simulink model "DataCenterStability"  (R2025b)
settings: Solver=daessc  StartTime=0  StopTime=7  FixedStep=5e-5  MaxStep=0.001  RelTol=1e-3
PostLoadFcn:
  | DataCenterParamScan
InitFcn:
  | opFile_ = fullfile(fileparts(which('DataCenterStability')), 'DataCenterStability_SteadyStateOP.mat');
  | if isfile(opFile_)
  |     tmp_ = load(opFile_, 'op');
  |     assignin('base', 'ssOP__', tmp_.op);
  | end
  | warning('off','physmod:common:mf:system:xform:DelayUnsupportedWithOperatingPoint');
  | warning('off','physmod:common:mf:system:xform:TimeUnsupportedWithOperatingPoint');
values from neighbouring files (symbols this model uses):
  baseVoltageDC = ups.Vdc    [DataCenterParamScan.m]
  bessConverterEfficiency = ups.DCBus.converterEff    [DataCenterParamScan.m]
  droopGain = ups.DCBus.droop    [DataCenterParamScan.m]
  filterInductance = ups.inverter.filterInductance    [DataCenterParamScan.m]
  filterInductanceAFE = ups.AFE.filterInductance    [DataCenterParamScan.m]
  filterResistance = ups.inverter.filterResistance    [DataCenterParamScan.m]
  filterResistanceAFE = ups.AFE.filterResistance    [DataCenterParamScan.m]
  frequency = ups.frequency    [DataCenterParamScan.m]
  G1 = 1    [DataCenterParamScan.m]
  G2 = 0    [DataCenterParamScan.m]
  iBatt = ups.batt.iRated    [DataCenterParamScan.m]
  initialMode = ups.batt.initialMode    [DataCenterParamScan.m]
  invKiId = ups.inverter.kiId    [DataCenterParamScan.m]
  invKiVd = ups.inverter.kiVd    [DataCenterParamScan.m]
  invKpId = ups.inverter.kpId    [DataCenterParamScan.m]
  invKpVd = ups.inverter.kpVd    [DataCenterParamScan.m]
  kpDC = ups.DCBus.kpDC    [DataCenterParamScan.m]
  N_pfc = round(N_total * [1/3, 1/3, 1/3])    [DataCenterParamScan.m]    (also in StabilityStudy.m = cfg.Topology.N_pfc)
  plantRating = ups.rating    [DataCenterParamScan.m]
  powerTau = 0.005    [DataCenterParamScan.m]
  rampRate = ups.batt.rampRate    [DataCenterParamScan.m]
  scan = obj.Cfg.GNC    [GNCAnalyzer.m]
  Ts = 5e-5    (= 5e-05)    [DataCenterParamScan.m]
  Vac = ups.Vac    [DataCenterParamScan.m]
  vBattMax = ups.batt.VMax    [DataCenterParamScan.m]
  vBattNom = ups.batt.Vnom    [DataCenterParamScan.m]
  vDCThreshold = ups.DCBus.VThreshold    [DataCenterParamScan.m]
  vGridMin = ups.DCBus.gridThreshold    [DataCenterParamScan.m]
undefined symbols (not defined in the file or in its folder): ctLimitDelayTime, DiscIntNeverNeededParam, ee_sli_rtmsupport, gcbh, itTray, pfc, serverTray, ups
libraries: fl_lib x77, nesl_utility x35, ee_lib x30, simulink x17, eeGeneralControl x14, datacenter_lib x12, eeTransforms x7, slpidlib x4, nesl_utility_internal x4, simulink_extras x3, datacenterCompositeLib x2, eePowerMeasurement x2
(part 1 of 5)
settings Model: SimulationMode=accelerator  Creator=rajarshd  LastModifiedBy=rajarshd
settings SolverCC: AllowMultiTaskInputOutput=on  ZeroCrossAlgorithm=Adaptive  AutoInsertRateTranBlk=on
settings DataIOCC: FinalStateName=xFinal_ss  InitialState=xInitOP__  SaveOperatingPoint=on  SaveOutput=off  DSMLogging=off  SaveTime=off  StateSaveName=xoutState
settings DebuggingCC: InheritedTsInSrcMsg=none  MultiTaskRateTransMsg=warning
settings SimscapeCC: SimscapeNominalValues="[{\"value\":\"1\",\"unit\":\"A\"},{\"value\":\"1\",\"unit\":\"bar\"},{\"value\":\"1\",\"unit\":\"cm^2\"},{\"value\":\"1\",\"unit\":\"cm^3/s\"},{\"value\":\"1\",\"unit\":\"kJ/kg\"},{\"value\":\"1\",\"unit\":\"kW\"},{\"value\":\"1\",\"unit\":\"l\"},{\"value\":\"1\",\"unit\":\"N\"},{\"value\":\"1\",\"unit\":\"N*m\"},{\"value\":\"1\",\"unit\":\"V\"},{\"value\":\"0.001\",\"unit\":\"Wb\"}]"  SimscapeLogType=all  SimscapeLogDecimation=50.0  SimscapeLogLimitData=off  SimscapeLogDataHistory=10000.0  SimscapeUseOperatingPoints=on  SimscapeOperatingPoint=ssOP__  SimscapeCompileComponentReuse=on
settings ExplorerConfigSet: SimMechanicsOpenEditorOnUpdate=off

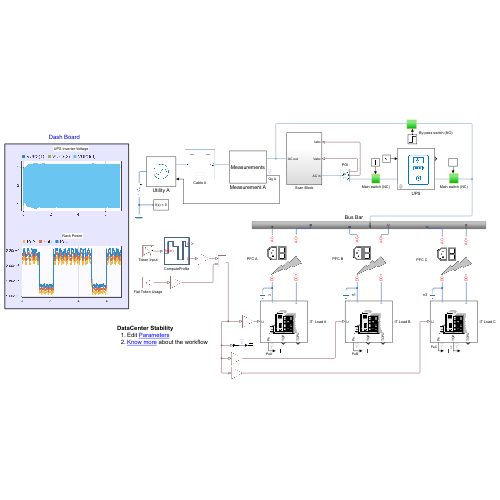
[thumbnail: Simulink's stored preview of the top-level diagram]
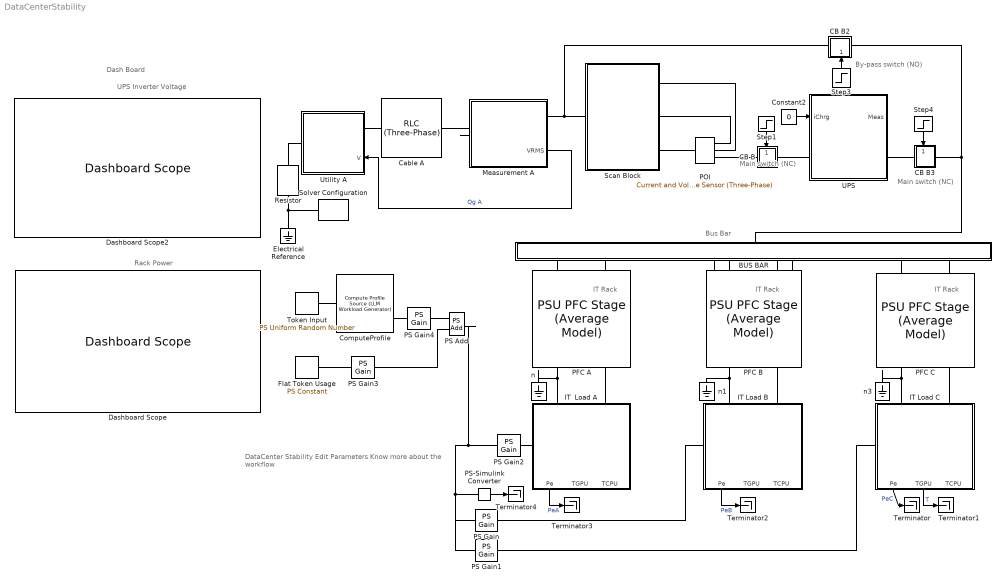
== system DataCenterStability ==
  note: DataCenter Stability
      | Edit Parameters
      | Know more about the workflow
  note: Dash Board
  note: By-pass switch (NO)
  note: Rack Power
  note: IT Rack
  note: IT Rack
  note: IT Rack
  note: Bus Bar
  note: Main switch (NC)
  note: Main switch (NC)
  note: UPS Inverter Voltage
  BUS BAR : Subsystem
  CB B : Subsystem
      settings: PortSchema="{\"entries\":[{\"content\":{\"sides\":[{\"content\":{\"connectorIds\":[\"In1\"]},\"type\":\"ConnectorPlacement.EquallySpacedRectSide\",\"uuid\":\"67c0f727-7c15-41c9-98df-b3c7d57498ed\"},{\"content\":{\"side\":\"RIGHT\"},\"type\":\"ConnectorPlacement.EquallySpacedRectSide\",\"uuid\":\"7fc39429-ba61-416d-b42b-93e81eb2f426\"},{\"content\":{\"connectorIds\":[\"LConn1\"],\"side\":\"TOP\"},\"type\":\"ConnectorPlacement.EquallySpacedRectSide\",\"uuid\":\"c6dd9263-b57a-4cff-a218-af99f2798f29\"},{\"content\":{\"connectorIds\":[\"RConn1\"],\"side\":\"BOTTOM\"},\"type\":\"ConnectorPlacement.EquallySpacedRectSide\",\"uuid\":\"e2a2ba44-d59d-4e27-adf1-3f94e828ca78\"}]},\"type\":\"ConnectorPlacement.EquallySpacedConnector\",\"uuid\":\"b349a99b-c902-4df9-9c99-34841afb28dd\"}],\"packageUris\":[\"http://schema.mathworks.com/mf0/Connector/R2020b\"],\"version\":\"1.0\"}"
  CB B2 : Subsystem
      settings: PortSchema="{\"entries\":[{\"content\":{\"sides\":[{\"content\":{},\"type\":\"ConnectorPlacement.EquallySpacedRectSide\",\"uuid\":\"67c0f727-7c15-41c9-98df-b3c7d57498ed\"},{\"content\":{\"connectorIds\":[\"In1\"],\"side\":\"RIGHT\"},\"type\":\"ConnectorPlacement.EquallySpacedRectSide\",\"uuid\":\"7fc39429-ba61-416d-b42b-93e81eb2f426\"},{\"content\":{\"connectorIds\":[\"LConn1\"],\"side\":\"TOP\"},\"type\":\"ConnectorPlacement.EquallySpacedRectSide\",\"uuid\":\"c6dd9263-b57a-4cff-a218-af99f2798f29\"},{\"content\":{\"connectorIds\":[\"RConn1\"],\"side\":\"BOTTOM\"},\"type\":\"ConnectorPlacement.EquallySpacedRectSide\",\"uuid\":\"e2a2ba44-d59d-4e27-adf1-3f94e828ca78\"}]},\"type\":\"ConnectorPlacement.EquallySpacedConnector\",\"uuid\":\"b349a99b-c902-4df9-9c99-34841afb28dd\"}],\"packageUris\":[\"http://schema.mathworks.com/mf0/Connector/R2020b\"],\"version\":\"1.0\"}"
  CB B3 : Subsystem
      settings: PortSchema="{\"entries\":[{\"content\":{\"sides\":[{\"content\":{\"connectorIds\":[\"In1\"]},\"type\":\"ConnectorPlacement.EquallySpacedRectSide\",\"uuid\":\"67c0f727-7c15-41c9-98df-b3c7d57498ed\"},{\"content\":{\"side\":\"RIGHT\"},\"type\":\"ConnectorPlacement.EquallySpacedRectSide\",\"uuid\":\"7fc39429-ba61-416d-b42b-93e81eb2f426\"},{\"content\":{\"connectorIds\":[\"LConn1\"],\"side\":\"TOP\"},\"type\":\"ConnectorPlacement.EquallySpacedRectSide\",\"uuid\":\"c6dd9263-b57a-4cff-a218-af99f2798f29\"},{\"content\":{\"connectorIds\":[\"RConn1\"],\"side\":\"BOTTOM\"},\"type\":\"ConnectorPlacement.EquallySpacedRectSide\",\"uuid\":\"e2a2ba44-d59d-4e27-adf1-3f94e828ca78\"}]},\"type\":\"ConnectorPlacement.EquallySpacedConnector\",\"uuid\":\"b349a99b-c902-4df9-9c99-34841afb28dd\"}],\"packageUris\":[\"http://schema.mathworks.com/mf0/Connector/R2020b\"],\"version\":\"1.0\"}"
  Cable A : ee_lib/Passive/RLC Assemblies/RLC (Three-Phase)  port_option=ee.enum.threePhasePort.composite  component_structure=ee.enum.rlc.structure.SeriesRL  R=0.001 Ohm  L=0.001 mH  C=1e-6 F  R_parasitic=0 Ohm  G_parasitic=0 1/Ohm  IL_specify=off  IL_priority=High  IL=[0, 0, 0] A  IL_nominal_specify=off  IL_nominal_value=1  IL_nominal_unit=A  VC_specify=off  VC_priority=High  VC=[0, 0, 0] V  VC_nominal_specify=off  VC_nominal_value=1  VC_nominal_unit=V
      settings: InternalSimscapePortConfiguration="{\"Bottom\":[],\"Left\":[{\"id\":\"N1\",\"label\":\"~1\",\"type\":\"foundation.electrical.three_phase\"}],\"Right\":[{\"id\":\"N2\",\"label\":\"~2\",\"type\":\"foundation.electrical.three_phase\"}],\"Top\":[]}"
  ComputeProfile : datacenter_lib/Compute Profile Source (LLM Workload Generator)  gpuModel=GPUModel.B200  numGPUs=numGPUs  workloadType=WorkloadType.Training  timeScale=4  tokenSource=TokenSource.Fixed  showAdvanced=true  customPeakTFLOPS=1000  customHbmBW=4e12 1/s  hbmBW=8e12 1/s  interNodeBW=50e9 1/s  llmSize=LLMModelSize.GPT_175B  customNumParams_B=70  customNumLayers=80  customPrecision=2  parallelism=ParallelismStrategy.TP8_PP4  customTP=8  customPP=4  microBatch=8  globalBatch=12288  seqLength=2048  idleUtil=0.60  fwdUtil=0.92  bwdUtil=0.98  commSyncUtil=0.65  prompt_tokens=512  output_tokens=256  num_concurrent=8  batch_size=8  allreduce_latency=5e-6 s  baseInfUtil=0.08  baseInfFrac=0.10  MFU=0.85  checkpointOverhead=0.03  stragglerOverhead=0.02  trainableParamFrac=0.02  evalInterval=5  evalBatches=2  ft_checkpointOverhead=0.05  enableNoise=true  noiseAmplitude=0.05  stepJitter=0  enableFilter=false  filterTimeConstant=0.01 s  t_step_specify=off  t_step_priority=Low  t_step=0 s  t_step_nominal_specify=off  t_step_nominal_value=1  t_step_nominal_unit=s  phase_id_specify=off  phase_id_priority=None  phase_id=0  phase_id_nominal_specify=off  phase_id_nominal_value=1  phase_id_nominal_unit=1  utilization_specify=off  utilization_priority=None  utilization=0  utilization_nominal_specify=off  utilization_nominal_value=1  utilization_nominal_unit=1  step_count_specify=off  step_count_priority=None  step_count=0  step_count_nominal_specify=off  step_count_nominal_value=1  step_count_nominal_unit=1  tc_utilization_specify=off  tc_utilization_priority=None  tc_utilization=0  tc_utilization_nominal_specify=off  tc_utilization_nominal_value=1  tc_utilization_nominal_unit=1  hbm_utilization_specify=off  hbm_utilization_priority=None  hbm_utilization=0  hbm_utilization_nominal_specify=off  hbm_utilization_nominal_value=1  hbm_utilization_nominal_unit=1  tokens_per_sec_obs_specify=off  tokens_per_sec_obs_priority=None  tokens_per_sec_obs=0 1/s  tokens_per_sec_obs_nominal_specify=off  tokens_per_sec_obs_nominal_value=1  tokens_per_sec_obs_nominal_unit=1/s  ttft_obs_specify=off  ttft_obs_priority=None  ttft_obs=0 s  ttft_obs_nominal_specify=off  ttft_obs_nominal_value=1  ttft_obs_nominal_unit=s
      settings: InternalSimscapePortConfiguration="{\"Bottom\":[],\"Left\":[{\"id\":\"prompt_len_in\",\"label\":\"Tn(in)\",\"type\":\"input\"}],\"Right\":[{\"id\":\"compute\",\"label\":\"C\",\"type\":\"output\"},{\"id\":\"U\",\"label\":\"U\",\"type\":\"output\"}],\"Top\":[]}"
  Constant2 : Constant  Value=0
  Dashboard Scope : DashboardScope  FontColor=[0.0, 0.0, 0.0]
  Dashboard Scope2 : DashboardScope  FontColor=[0.0, 0.0, 0.0]
  Electrical Reference : fl_lib/Electrical/Electrical Elements/Electrical Reference
  Flat Token Usage : fl_lib/Physical Signals/Sources/PS Constant  constant=0.5
  IT  Load A : Subsystem
      settings: PortSchema="{\"entries\":[{\"content\":{\"sides\":[{\"content\":{\"connectorIds\":[\"LConn1\",\"LConn2\"]},\"type\":\"ConnectorPlacement.EquallySpacedRectSide\",\"uuid\":\"2a986be5-1ee0-42f2-ba1d-7e7b19b6aff8\"},{\"content\":{\"connectorIds\":[\"Out1\",\"Out2\",\"Out3\"],\"side\":\"RIGHT\"},\"type\":\"ConnectorPlacement.EquallySpacedRectSide\",\"uuid\":\"6fb5a5ce-a365-4ece-bf73-56d3378d5391\"},{\"content\":{\"connectorIds\":[\"LConn3\"],\"side\":\"TOP\"},\"type\":\"ConnectorPlacement.EquallySpacedRectSide\",\"uuid\":\"7ef05e6e-a854-4441-a4de-558238083686\"}]},\"type\":\"ConnectorPlacement.EquallySpacedConnector\",\"uuid\":\"2a3433b7-bc52-494b-97a4-7ef9d11a25e3\"}],\"packageUris\":[\"http://schema.mathworks.com/mf0/Connector/R2020b\"],\"version\":\"1.0\"}"
      mask Display: image('datacenter.png', [0,0,0,0,80,80]);
  IT Load B : Subsystem
      settings: PortSchema="{\"entries\":[{\"content\":{\"sides\":[{\"content\":{\"connectorIds\":[\"LConn1\",\"LConn2\"]},\"type\":\"ConnectorPlacement.EquallySpacedRectSide\",\"uuid\":\"2a986be5-1ee0-42f2-ba1d-7e7b19b6aff8\"},{\"content\":{\"connectorIds\":[\"Out1\",\"Out2\",\"Out3\"],\"side\":\"RIGHT\"},\"type\":\"ConnectorPlacement.EquallySpacedRectSide\",\"uuid\":\"6fb5a5ce-a365-4ece-bf73-56d3378d5391\"},{\"content\":{\"connectorIds\":[\"LConn3\"],\"side\":\"TOP\"},\"type\":\"ConnectorPlacement.EquallySpacedRectSide\",\"uuid\":\"7ef05e6e-a854-4441-a4de-558238083686\"}]},\"type\":\"ConnectorPlacement.EquallySpacedConnector\",\"uuid\":\"2a3433b7-bc52-494b-97a4-7ef9d11a25e3\"}],\"packageUris\":[\"http://schema.mathworks.com/mf0/Connector/R2020b\"],\"version\":\"1.0\"}"
      mask Display: image('datacenter.png', [0,0,0,0,80,80]);
  IT Load C : Subsystem
      settings: PortSchema="{\"entries\":[{\"content\":{\"sides\":[{\"content\":{\"connectorIds\":[\"LConn1\",\"LConn2\"]},\"type\":\"ConnectorPlacement.EquallySpacedRectSide\",\"uuid\":\"2a986be5-1ee0-42f2-ba1d-7e7b19b6aff8\"},{\"content\":{\"connectorIds\":[\"Out1\",\"Out2\",\"Out3\"],\"side\":\"RIGHT\"},\"type\":\"ConnectorPlacement.EquallySpacedRectSide\",\"uuid\":\"6fb5a5ce-a365-4ece-bf73-56d3378d5391\"},{\"content\":{\"connectorIds\":[\"LConn3\"],\"side\":\"TOP\"},\"type\":\"ConnectorPlacement.EquallySpacedRectSide\",\"uuid\":\"7ef05e6e-a854-4441-a4de-558238083686\"}]},\"type\":\"ConnectorPlacement.EquallySpacedConnector\",\"uuid\":\"2a3433b7-bc52-494b-97a4-7ef9d11a25e3\"}],\"packageUris\":[\"http://schema.mathworks.com/mf0/Connector/R2020b\"],\"version\":\"1.0\"}"
      mask Display: image('datacenter.png', [0,0,0,0,80,80]);
  Measurement A : Subsystem
      settings: PortSchema="{\"entries\":[{\"content\":{\"sides\":[{\"content\":{\"connectorIds\":[\"LConn1\"]},\"type\":\"ConnectorPlacement.EquallySpacedRectSide\",\"uuid\":\"eb9abe54-d1fe-49de-8ced-a6e10c1202db\"},{\"content\":{\"connectorIds\":[\"RConn1\",\"Out1\"],\"side\":\"RIGHT\"},\"type\":\"ConnectorPlacement.EquallySpacedRectSide\",\"uuid\":\"002de1fc-31bd-4798-a6dd-d6b957f4e96f\"},{\"content\":{\"side\":\"TOP\"},\"type\":\"ConnectorPlacement.EquallySpacedRectSide\",\"uuid\":\"be5aa959-f6e3-4875-a946-227b594aa2c5\"}]},\"type\":\"ConnectorPlacement.EquallySpacedConnector\",\"uuid\":\"8ade2fe3-03c6-4466-8b3c-15c4c721ac97\"}],\"packageUris\":[\"http://schema.mathworks.com/mf0/Connector/R2020b\"],\"version\":\"1.0\"}"
      mask Display: disp('Measurements');
  PFC A : datacenter_lib/PSU PFC Stage (Average Model)  C_dc=3.99 F  V_dc_ref=pfc.V_dc_ref V  Kp_pfc=26600 W/V  Ki_pfc=79800 W/(V*s)  eta_pfc=pfc.eta  P_max=N_pfc(1) * pfc.P_max MW  G_damp=0.266 1/Ohm  tau_rms=pfc.tau_rms s  V_nom=pfc.V_nom V  L_ac=pfc.L_ac / N_pfc(1) H  R_ac=pfc.R_ac / N_pfc(1) Ohm  i_ac_specify=off  i_ac_priority=None  i_ac=0 A  i_ac_nominal_specify=off  i_ac_nominal_value=1  i_ac_nominal_unit=A  v_ac_specify=off  v_ac_priority=Low  v_ac=277 V  v_ac_nominal_specify=off  v_ac_nominal_value=1  v_ac_nominal_unit=V  v_dc_specify=on  v_dc_priority=High  v_dc=400 V  v_dc_nominal_specify=off  v_dc_nominal_value=1  v_dc_nominal_unit=V  i_dc_specify=off  i_dc_priority=None  i_dc=0 A  i_dc_nominal_specify=off  i_dc_nominal_value=1  i_dc_nominal_unit=A  pfc_integrator_specify=on  pfc_integrator_priority=Low  pfc_integrator=0 V*s  pfc_integrator_nominal_specify=off  pfc_integrator_nominal_value=1  pfc_integrator_nominal_unit=V*s  v_rms_sq_specify=off  v_rms_sq_priority=Low  v_rms_sq=76729 V^2  v_rms_sq_nominal_specify=off  v_rms_sq_nominal_value=1  v_rms_sq_nominal_unit=V^2
      settings: InternalSimscapePortConfiguration="{\"Bottom\":[],\"Left\":[{\"id\":\"p\",\"label\":\"AC+\",\"type\":\"foundation.electrical.electrical\"},{\"id\":\"n\",\"label\":\"AC-\",\"type\":\"foundation.electrical.electrical\"}],\"Right\":[{\"id\":\"dc_p\",\"label\":\"DC+\",\"type\":\"foundation.electrical.electrical\"},{\"id\":\"dc_n\",\"label\":\"DC-\",\"type\":\"foundation.electrical.electrical\"}],\"Top\":[]}"
  PFC B : datacenter_lib/PSU PFC Stage (Average Model)  C_dc=3.99 F  V_dc_ref=pfc.V_dc_ref V  Kp_pfc=26600 W/V  Ki_pfc=79800 W/(V*s)  eta_pfc=pfc.eta  P_max=N_pfc(2) * pfc.P_max MW  G_damp=0.266 1/Ohm  tau_rms=pfc.tau_rms s  V_nom=pfc.V_nom V  L_ac=pfc.L_ac / N_pfc(2) H  R_ac=pfc.R_ac / N_pfc(2) Ohm  i_ac_specify=off  i_ac_priority=None  i_ac=0 A  i_ac_nominal_specify=off  i_ac_nominal_value=1  i_ac_nominal_unit=A  v_ac_specify=off  v_ac_priority=Low  v_ac=277 V  v_ac_nominal_specify=off  v_ac_nominal_value=1  v_ac_nominal_unit=V  v_dc_specify=on  v_dc_priority=High  v_dc=400 V  v_dc_nominal_specify=off  v_dc_nominal_value=1  v_dc_nominal_unit=V  i_dc_specify=off  i_dc_priority=None  i_dc=0 A  i_dc_nominal_specify=off  i_dc_nominal_value=1  i_dc_nominal_unit=A  pfc_integrator_specify=on  pfc_integrator_priority=Low  pfc_integrator=0 V*s  pfc_integrator_nominal_specify=off  pfc_integrator_nominal_value=1  pfc_integrator_nominal_unit=V*s  v_rms_sq_specify=off  v_rms_sq_priority=Low  v_rms_sq=76729 V^2  v_rms_sq_nominal_specify=off  v_rms_sq_nominal_value=1  v_rms_sq_nominal_unit=V^2
      settings: InternalSimscapePortConfiguration="{\"Bottom\":[],\"Left\":[{\"id\":\"p\",\"label\":\"AC+\",\"type\":\"foundation.electrical.electrical\"},{\"id\":\"n\",\"label\":\"AC-\",\"type\":\"foundation.electrical.electrical\"}],\"Right\":[{\"id\":\"dc_p\",\"label\":\"DC+\",\"type\":\"foundation.electrical.electrical\"},{\"id\":\"dc_n\",\"label\":\"DC-\",\"type\":\"foundation.electrical.electrical\"}],\"Top\":[]}"
  PFC C : datacenter_lib/PSU PFC Stage (Average Model)  C_dc=4.02 F  V_dc_ref=pfc.V_dc_ref V  Kp_pfc=26800 W/V  Ki_pfc=80400 W/(V*s)  eta_pfc=pfc.eta  P_max=N_pfc(3) * pfc.P_max MW  G_damp=0.268 1/Ohm  tau_rms=pfc.tau_rms s  V_nom=pfc.V_nom V  L_ac=pfc.L_ac / N_pfc(3) H  R_ac=pfc.R_ac / N_pfc(3) Ohm  i_ac_specify=off  i_ac_priority=None  i_ac=0 A  i_ac_nominal_specify=off  i_ac_nominal_value=1  i_ac_nominal_unit=A  v_ac_specify=off  v_ac_priority=Low  v_ac=277 V  v_ac_nominal_specify=off  v_ac_nominal_value=1  v_ac_nominal_unit=V  v_dc_specify=on  v_dc_priority=High  v_dc=400 V  v_dc_nominal_specify=off  v_dc_nominal_value=1  v_dc_nominal_unit=V  i_dc_specify=off  i_dc_priority=None  i_dc=0 A  i_dc_nominal_specify=off  i_dc_nominal_value=1  i_dc_nominal_unit=A  pfc_integrator_specify=on  pfc_integrator_priority=Low  pfc_integrator=0 V*s  pfc_integrator_nominal_specify=off  pfc_integrator_nominal_value=1  pfc_integrator_nominal_unit=V*s  v_rms_sq_specify=off  v_rms_sq_priority=Low  v_rms_sq=76729 V^2  v_rms_sq_nominal_specify=off  v_rms_sq_nominal_value=1  v_rms_sq_nominal_unit=V^2
      settings: InternalSimscapePortConfiguration="{\"Bottom\":[],\"Left\":[{\"id\":\"p\",\"label\":\"AC+\",\"type\":\"foundation.electrical.electrical\"},{\"id\":\"n\",\"label\":\"AC-\",\"type\":\"foundation.electrical.electrical\"}],\"Right\":[{\"id\":\"dc_p\",\"label\":\"DC+\",\"type\":\"foundation.electrical.electrical\"},{\"id\":\"dc_n\",\"label\":\"DC-\",\"type\":\"foundation.electrical.electrical\"}],\"Top\":[]}"
  POI : ee_lib/Sensors & Transducers/Current and Voltage Sensor (Three-Phase)  vMeasurementType=ee.enum.vmeasurement.lg  outputUnit=ee.enum.unit.si  SRated=1e6 A*V  VRated=base.kV V  I_specify=off  I_priority=None  I=[0, 0, 0] A  I_nominal_specify=off  I_nominal_value=1  I_nominal_unit=A  V_specify=off  V_priority=None  V=[0, 0, 0] V  V_nominal_specify=off  V_nominal_value=1  V_nominal_unit=V
      settings: InternalSimscapePortConfiguration="{\"Bottom\":[],\"Left\":[{\"id\":\"N1\",\"label\":\"~1\",\"type\":\"foundation.electrical.three_phase\"}],\"Right\":[{\"id\":\"V_output\",\"label\":\"V\",\"type\":\"output\"},{\"id\":\"I_output\",\"label\":\"I\",\"type\":\"output\"},{\"id\":\"N2\",\"label\":\"~2\",\"type\":\"foundation.electrical.three_phase\"}],\"Top\":[]}"
  PS Add : fl_lib/Physical Signals/Functions/PS Add
  PS Gain : fl_lib/Physical Signals/Functions/PS Gain  gain=0.95
  PS Gain1 : fl_lib/Physical Signals/Functions/PS Gain  gain=1
  PS Gain2 : fl_lib/Physical Signals/Functions/PS Gain  gain=0.9
  PS Gain3 : fl_lib/Physical Signals/Functions/PS Gain  gain=G2
  PS Gain4 : fl_lib/Physical Signals/Functions/PS Gain  gain=G1
  PS-Simulink Converter : nesl_utility/PS-Simulink Converter  PhysicalDomain=network_engine_domain  SubClassName=ps_output  LeftPortType=input  RightPortType=output  PseudoPeriodic=off  Frequencies=[]  VectorFormat=inherit  Unit=inherit  AffineConversion=off
  Resistor : fl_lib/Electrical/Electrical Elements/Resistor  R=1e-6 Ohm  i_specify=off  i_priority=None  i=0 A  i_nominal_specify=off  i_nominal_value=1  i_nominal_unit=A  v_specify=off  v_priority=None  v=0 V  v_nominal_specify=off  v_nominal_value=1  v_nominal_unit=V
  Scan Block : Subsystem
  Solver Configuration : nesl_utility/Solver Configuration  PhysicalDomain=network_engine_domain  SubClassName=solver  LeftPortType=input  RightPortType=generic  Tones=[]  Harmonics=[]  SimulateNoise=off  Profile=off  UseLocalSampling=off  EnableSwitchedLinearOptims=on  FrequencyDomain=off  UseCCode=off  RelTol=0.001  AbsTol=0.001  MinStep=1e-09  ToWorkspace=off  RevertToSquareIcSolve=off  NumHomotopyIterations=100  PhasorMode=off  PhasorModeNumHarmonics=1  ConsistencySolver=NEWTON_XTOL_AFTER_FTOL  IndexReductionMethod=None  DoDC=off  ResidualTolerance=1e-6  ConsistencyTolSource=LOCAL  ConsistencyAbsTol=1e3  ConsistencyRelTol=1e3  ConsistencyTolFactor=1e3  UseLocalSolver=on  LocalSolverChoice=NE_BACKWARD_EULER_ADVANCER  ResolveIndetEquations=off  FunctionEvalNumThread=1  LocalSolverSampleTime=5e-05  DoFixedCost=on  MaxNonlinIter=1  MaxModeIter=2  ComputeImpulses=off  ImpulseIterations=2  LinearAlgebra=Sparse  LinearAlgebraNumThread=0  EquationFormulation=NE_TIME_EF  DelaysMemoryBudget=1024  AutomaticFiltering=off  FilteringTimeConstant=0.001  PartitionStorageMethod=AS_NEEDED  PartitionMemoryBudget=1024  PartitionMethod=ROBUST  MultibodyUseLocalSolver=off  MultibodyLocalSolverChoice=ODE1  MultibodyLocalSolverSampleTime=0.001
  Step1 : Step  Time=0  After=0  SampleTime=1e-4
  Step3 : Step  Time=0  Before=1  SampleTime=1e-4
  Step4 : Step  Time=0  After=0  SampleTime=1e-4
  Terminator{,1..4} (5 alike) : Terminator
  Token Input : fl_lib/Physical Signals/Sources/PS Uniform Random Number  minimum=1  maximum=10  initial_seed=0  sample_time=Ts s
      settings: InternalSimscapePortConfiguration="{\"Bottom\":[],\"Left\":[],\"Right\":[{\"id\":\"Y\",\"label\":\"Y\",\"type\":\"output\"}],\"Top\":[]}"
  UPS : Subsystem  VariantControl=Detailed  mask(Double-conversion Uniterrupted Power Supply (UPS)){plantRating=plantRating, Vac=Vac, frequency=frequency, baseVoltageDC=baseVoltageDC, sampleTime=ups.sampleTime, filterInductanceAFE=filterInductanceAFE, filterResistanceAFE=filterResistanceAFE, capacitance=1.6, vBattNom=vBattNom, iBatt=iBatt, vBattMax=vBattMax, droopGain=droopGain, rampRate=rampRate, vGridMin=vGridMin, vDCThreshold=vDCThreshold, initialMode=initialMode, kpDC=kpDC, kiDC=1200, bessConverterEfficiency=bessConverterEfficiency, filterInductance=filterInductance, filterResistance=filterResistance, invKpVd=invKpVd, invKiVd=invKiVd, invKpId=invKpId, invKiId=invKiId}
      mask prompts: plantRating "UPS Rating (kW)"; Vac "Rated AC side voltage (phase-phase RMS) (V)"; frequency "Rated electrical frequency at AC side (Hz)"; baseVoltageDC "Voltage on DC side (V)"; sampleTime "Sample time (s)"; filterInductanceAFE "Filter inductance (H)"; filterResistanceAFE "Filter resistance (Ohm)"; capacitance "Capacitance (F)"; vBattNom "Battery nominal voltage (V)"; iBatt "Battery rated current (A)"; vBattMax "Maximum battery voltage (V)"; droopGain "DC bus droop gain"; rampRate "Ramp rate for battery discharge"; vGridMin "Minimum grid voltage (V)"; vDCThreshold "Threshold DC Bus voltage (V)"; initialMode "Initial operating mode"; kpDC "DC-DC Converter proportional gain"; kiDC "DC-DC Converter integral gain"; bessConverterEfficiency "DC-DC converter efficiency (%)"; filterInductance "Filter inductance (H)"; filterResistance "Filter series resistance (Ohm)"; invKpVd "Inverter Kp Vd"; invKiVd "Inverter Ki Vd"; invKpId "Inverter Kp Id"; invKiId "Inverter Ki Id"
      mask help: This block models a double conversion uninterruptible power supply that continuously supplies the load through an inverter. It isolates the load from input disturbances and uses a battery on the DC link to maintain uninterrupted power during input outages.
      mask Help: web('UPS.html')
      mask DialogControl generalDetailed Prompt: General
      mask DialogControl Container9 Prompt: Active Front End
      mask DialogControl editRectifier Prompt: Edit converter parameters
      mask DialogControl editRectifier Callback:
      | blockPath = [gcb,'/','Rectifier','/','AC-DC Converter'];
      |     component.mask.openBlock(blockPath);
      mask DialogControl configureAFEController Prompt: Edit AFE controller
      mask DialogControl configureAFEController Callback:
      | blockPath = [gcb,'/','Rectifier','/','PFC Rectifier Controller'];
      |     component.mask.openBlock(blockPath);
      mask DialogControl cellDetailed Prompt: DC Link
      mask DialogControl configureBattery Prompt: Edit battery parameters
      mask DialogControl configureBattery Callback:
      | blockPath = [gcb,'/','DC-Link','/','BESS','/','Battery'] ;
      |     component.mask.openBlock(blockPath);
      mask DialogControl controllerDetailed Prompt: Inverter
      mask DialogControl editInverter Prompt: Edit converter parameters
      mask DialogControl editInverter Callback:
      | blockPath = [gcb,'/','Inverter','/','DC- AC Converter'];
      |     component.mask.openBlock(blockPath);
      mask DialogControl editInverterController Prompt: Edit inverter controller
      mask DialogControl editInverterController Callback:
      | blockPath = [gcb,'/','Inverter','/','Inverter Controller'] ;
      |     component.mask.openBlock(blockPath);
  Utility A : Subsystem
      settings: PortSchema="{\"entries\":[{\"content\":{\"sides\":[{\"content\":{\"connectorIds\":[\"LConn1\",\"In1\"]},\"type\":\"ConnectorPlacement.EquallySpacedRectSide\",\"uuid\":\"d3f99cc1-1428-452a-9ffe-24ae0795f56a\"},{\"content\":{\"connectorIds\":[\"RConn1\"],\"side\":\"RIGHT\"},\"type\":\"ConnectorPlacement.EquallySpacedRectSide\",\"uuid\":\"01ef32cb-94a8-4968-996d-9de41577beb5\"},{\"content\":{\"side\":\"TOP\"},\"type\":\"ConnectorPlacement.EquallySpacedRectSide\",\"uuid\":\"ffdd87d9-752e-49dd-9088-d01f0a2a90f0\"}]},\"type\":\"ConnectorPlacement.EquallySpacedConnector\",\"uuid\":\"6becf236-9c53-43c5-89f8-133ab6ea3988\"}],\"packageUris\":[\"http://schema.mathworks.com/mf0/Connector/R2020b\"],\"version\":\"1.0\"}"
  n : fl_lib/Electrical/Electrical Elements/Electrical Reference
  n1 : fl_lib/Electrical/Electrical Elements/Electrical Reference
  n3 : fl_lib/Electrical/Electrical Elements/Electrical Reference
  wires:
  Constant2/1 -> UPS/1(iChrg)
  IT Load C/2(TGPU) -> Terminator1/1  "T"
  IT Load C/1(Pe) -> Terminator/1  "PeC"
  Step3/1 -> CB B2/1(input0)
  Step1/1 -> CB B/1(input0)
  Step4/1 -> CB B3/1(input0)
  IT Load B/1(Pe) -> Terminator2/1  "PeB"
  IT  Load A/1(Pe) -> Terminator3/1  "PeA"
  PS-Simulink Converter/1 -> Terminator4/1
  Measurement A/1(VRMS) -> Utility A/1(V)  "Qg A"
  connections:
  Resistor/LConn1 -- Utility A/RConn1
  Measurement A/LConn1 -- Cable A/RConn1
  Token Input/RConn1 -- ComputeProfile/LConn1
  Electrical Reference/LConn1 -- Solver Configuration/RConn1 -- Resistor/RConn1
  n/LConn1 -- IT  Load A/LConn1 -- PFC A/RConn2
  PFC B/RConn2 -- IT Load B/LConn1 -- n1/LConn1
  PFC A/LConn1 -- BUS BAR/RConn2
  PFC A/LConn2 -- BUS BAR/RConn1
  PFC B/LConn1 -- BUS BAR/RConn4
  PFC B/LConn2 -- BUS BAR/RConn3
  PFC C/LConn1 -- BUS BAR/RConn6
  PFC C/LConn2 -- BUS BAR/RConn5
  CB B2/RConn1 -- BUS BAR/LConn1 -- CB B3/RConn1
  IT Load C/LConn3 -- PS Gain1/RConn1
  IT Load B/LConn3 -- PS Gain/RConn1
  PS Gain2/RConn1 -- IT  Load A/LConn3
  IT  Load A/LConn2 -- PFC A/RConn1
  IT Load B/LConn2 -- PFC B/RConn1
  IT Load C/LConn2 -- PFC C/RConn1
  IT Load C/LConn1 -- n3/LConn1 -- PFC C/RConn2
  CB B/RConn1 -- UPS/LConn1
  CB B3/LConn1 -- UPS/RConn1
  Utility A/LConn1 -- Cable A/LConn1
  POI/LConn1 -- Scan Block/RConn3
  Measurement A/RConn1 -- CB B2/LConn1 -- Scan Block/LConn1
  POI/RConn3 -- CB B/LConn1
  POI/RConn2 -- Scan Block/RConn1
  POI/RConn1 -- Scan Block/RConn2
  PS Gain3/LConn1 -- Flat Token Usage/RConn1
  PS Gain4/LConn1 -- ComputeProfile/RConn2
  PS Add/LConn1 -- PS Gain4/RConn1
  PS Gain3/RConn1 -- PS Add/LConn2
  PS Add/RConn1 -- PS-Simulink Converter/LConn1 -- PS Gain1/LConn1 -- PS Gain/LConn1 -- PS Gain2/LConn1

== system DataCenterStability/BUS BAR ==
  Phase Splitter : ee_lib/Connectors & References/Phase Splitter
  Resistor : fl_lib/Electrical/Electrical Elements/Resistor  R=1e-4 Ohm  i_specify=off  i_priority=None  i=0 A  i_nominal_specify=off  i_nominal_value=1  i_nominal_unit=A  v_specify=off  v_priority=None  v=0 V  v_nominal_specify=off  v_nominal_value=1  v_nominal_unit=V
  Resistor1 : fl_lib/Electrical/Electrical Elements/Resistor  R=1e-6 Ohm  i_specify=off  i_priority=None  i=0 A  i_nominal_specify=off  i_nominal_value=1  i_nominal_unit=A  v_specify=off  v_priority=None  v=0 V  v_nominal_specify=off  v_nominal_value=1  v_nominal_unit=V
  Resistor2 : fl_lib/Electrical/Electrical Elements/Resistor  R=1e-6 Ohm  i_specify=off  i_priority=None  i=0 A  i_nominal_specify=off  i_nominal_value=1  i_nominal_unit=A  v_specify=off  v_priority=None  v=0 V  v_nominal_specify=off  v_nominal_value=1  v_nominal_unit=V
  abc : PMIOPort  Side=Left
  A : PMIOPort  Port=2  Side=Right
  ~B : PMIOPort  Port=3  Side=Right
  B : PMIOPort  Port=4  Side=Right
  ~C : PMIOPort  Port=5  Side=Right
  C : PMIOPort  Port=6  Side=Right
  ~A : PMIOPort  Port=7  Side=Right
  connections:
  abc/RConn1 -- Phase Splitter/LConn1
  Phase Splitter/RConn1 -- Resistor/LConn1 -- ~A/RConn1
  Phase Splitter/RConn2 -- ~B/RConn1 -- Resistor1/LConn1
  Resistor2/LConn1 -- Phase Splitter/RConn3 -- ~C/RConn1
  Resistor/RConn1 -- A/RConn1
  Resistor1/RConn1 -- B/RConn1
  Resistor2/RConn1 -- C/RConn1

== system DataCenterStability/CB B ==
  input0 : Inport
  Subsystem1 : Subsystem
      settings: PortSchema="{\"entries\":[{\"content\":{\"sides\":[{\"content\":{\"connectorIds\":[\"LConn1\",\"In1\"]},\"type\":\"ConnectorPlacement.EquallySpacedRectSide\",\"uuid\":\"4d523b2f-3490-490d-9193-0c3e52b1c3a1\"},{\"content\":{\"connectorIds\":[\"RConn1\"],\"side\":\"RIGHT\"},\"type\":\"ConnectorPlacement.EquallySpacedRectSide\",\"uuid\":\"1543a14a-65b5-4637-8d41-6da95a6ca307\"},{\"content\":{\"side\":\"TOP\"},\"type\":\"ConnectorPlacement.EquallySpacedRectSide\",\"uuid\":\"9fff8ee8-4727-466f-977a-681c4f14cc56\"}]},\"type\":\"ConnectorPlacement.EquallySpacedConnector\",\"uuid\":\"a46df766-bf17-4bd6-a8b3-579011040ee9\"}],\"packageUris\":[\"http://schema.mathworks.com/mf0/Connector/R2020b\"],\"version\":\"1.0\"}"
  Conn2 : PMIOPort  Side=Left
  in2 : PMIOPort  Port=2  Side=Right
  wires:
  input0/1 -> Subsystem1/1(input0)
  connections:
  Conn2/RConn1 -- Subsystem1/RConn1
  Subsystem1/LConn1 -- in2/RConn1

== system DataCenterStability/CB B2 ==
  input0 : Inport
  Subsystem1 : Subsystem
      settings: PortSchema="{\"entries\":[{\"content\":{\"sides\":[{\"content\":{\"connectorIds\":[\"LConn1\",\"In1\"]},\"type\":\"ConnectorPlacement.EquallySpacedRectSide\",\"uuid\":\"4d523b2f-3490-490d-9193-0c3e52b1c3a1\"},{\"content\":{\"connectorIds\":[\"RConn1\"],\"side\":\"RIGHT\"},\"type\":\"ConnectorPlacement.EquallySpacedRectSide\",\"uuid\":\"1543a14a-65b5-4637-8d41-6da95a6ca307\"},{\"content\":{\"side\":\"TOP\"},\"type\":\"ConnectorPlacement.EquallySpacedRectSide\",\"uuid\":\"9fff8ee8-4727-466f-977a-681c4f14cc56\"}]},\"type\":\"ConnectorPlacement.EquallySpacedConnector\",\"uuid\":\"a46df766-bf17-4bd6-a8b3-579011040ee9\"}],\"packageUris\":[\"http://schema.mathworks.com/mf0/Connector/R2020b\"],\"version\":\"1.0\"}"
  Conn2 : PMIOPort  Side=Left
  in2 : PMIOPort  Port=2  Side=Right
  wires:
  input0/1 -> Subsystem1/1(input0)
  connections:
  Conn2/RConn1 -- Subsystem1/RConn1
  Subsystem1/LConn1 -- in2/RConn1

== system DataCenterStability/CB B3 ==
  input0 : Inport
  Subsystem1 : Subsystem
      settings: PortSchema="{\"entries\":[{\"content\":{\"sides\":[{\"content\":{\"connectorIds\":[\"LConn1\",\"In1\"]},\"type\":\"ConnectorPlacement.EquallySpacedRectSide\",\"uuid\":\"4d523b2f-3490-490d-9193-0c3e52b1c3a1\"},{\"content\":{\"connectorIds\":[\"RConn1\"],\"side\":\"RIGHT\"},\"type\":\"ConnectorPlacement.EquallySpacedRectSide\",\"uuid\":\"1543a14a-65b5-4637-8d41-6da95a6ca307\"},{\"content\":{\"side\":\"TOP\"},\"type\":\"ConnectorPlacement.EquallySpacedRectSide\",\"uuid\":\"9fff8ee8-4727-466f-977a-681c4f14cc56\"}]},\"type\":\"ConnectorPlacement.EquallySpacedConnector\",\"uuid\":\"a46df766-bf17-4bd6-a8b3-579011040ee9\"}],\"packageUris\":[\"http://schema.mathworks.com/mf0/Connector/R2020b\"],\"version\":\"1.0\"}"
  Conn2 : PMIOPort  Side=Left
  in2 : PMIOPort  Port=2  Side=Right
  wires:
  input0/1 -> Subsystem1/1(input0)
  connections:
  Conn2/RConn1 -- Subsystem1/RConn1
  Subsystem1/LConn1 -- in2/RConn1

== system DataCenterStability/IT  Load A ==
  " IT Load" : ee_lib/Passive/Dynamic Load  load_type=ee.enum.dc_ac.dc  min_supply_voltage=0.5 V  pow_min=1e-3 W  G_reverse=1e-6 S  deltaV=1e-3 V  f0=60 Hz  Vrms_min=200 V  tau=0.01 s  Vrms_ini=300 V  Vang_ini=0 deg
      settings: InternalSimscapePortConfiguration="{\"Bottom\":[],\"Left\":[{\"id\":\"p\",\"label\":\"+\",\"type\":\"foundation.electrical.electrical\"}],\"Right\":[{\"id\":\"n\",\"label\":\"-\",\"type\":\"foundation.electrical.electrical\"}],\"Top\":[{\"id\":\"P\",\"label\":\"P\",\"type\":\"input\"}]}"
  Capacitor : fl_lib/Electrical/Electrical Elements/Capacitor  c=1e-3 F  r=1e-4 Ohm  g=1e-6 1/Ohm  i_specify=off  i_priority=None  i=0 A  i_nominal_specify=off  i_nominal_value=1  i_nominal_unit=A  v_specify=off  v_priority=None  v=0 V  v_nominal_specify=off  v_nominal_value=1  v_nominal_unit=V  vc_specify=on  vc_priority=Low  vc=400 V  vc_nominal_specify=off  vc_nominal_value=1  vc_nominal_unit=V
  Current Sensor : fl_lib/Electrical/Electrical Sensors/Current Sensor
  DC-DC Converter : ee_lib/Semiconductors & Converters/Converters/DC-DC Converter  Vref_option=ee.enum.converters.voltageref.internal  v_ref=1 V  P_rated=itTray.dcdc.P_rated(1) MW  droop_enabled=false  droop_param=ee.enum.converters.droop.value  droop=0.1 V/A  droop_percent=2  Vref_droop=10 V  reversible=ee.enum.converters.directionality.unidirectional  G_diode=1e-8 1/Ohm  P_fixed=1 W  losses_option=ee.enum.converters.lossesOption.proportionalToSquaredCurrent  eff_rated=itTray.dcdc.eff * 100  tableOption=ee.enum.converters.lossTableOptionThermal.currentTemp  i_eff_vec=[-2, -1, 1, 2] A  v_eff_vec=[15, 30, 45] V  eff_vec=[66, 76, 80, 74]  eff_2D_table=[66, 66, 66; 76, 76, 76; 80, 80, 80; 74, 74, 74]  model_dynamics=ee.enum.converters.dynamics.no  tau=0.02 s  v_ini=10 V  v1_min=1 V  R1=1000 Ohm  R2=1000 Ohm  fault_condition=ee.enum.faults.faultInputCondition.greaterThan  fault_threshold=0.5  T_eff_vec=[280, 300, 320] K  eff_3D_table=repmat([66; 76; 80; 74], 1, 3, 3)  thermal_mass=100 J/K  initial_temperature=298.15 K
      settings: InternalSimscapePortConfiguration="{\"Bottom\":[],\"Left\":[{\"id\":\"p1\",\"label\":\"1+\",\"type\":\"foundation.electrical.electrical\"},{\"id\":\"n1\",\"label\":\"1-\",\"type\":\"foundation.electrical.electrical\"}],\"Right\":[{\"id\":\"p2\",\"label\":\"2+\",\"type\":\"foundation.electrical.electrical\"},{\"id\":\"n2\",\"label\":\"2-\",\"type\":\"foundation.electrical.electrical\"},{\"id\":\"H\",\"label\":\"H\",\"type\":\"foundation.thermal.thermal\"}],\"Top\":[]}"
  Electrical Reference : fl_lib/Electrical/Electrical Elements/Electrical Reference
  PDU Racks : Subsystem  mask{nTrays=36, nRacks=6, trayMass=serverTray.trayMass, trayCp=serverTray.trayCp, trayThermalR=serverTray.trayThermalR_perGPU / itTray.nGPU(1), nGPU=itTray.nGPU(1), gpuTDPperDie=serverTray.gpuTDPperDie, gpuIdlePower=serverTray.gpuIdlePower, gpuHBMpower=serverTray.gpuHBMpower, gpuExponent=serverTray.gpuExponent, gpuHBMutil=serverTray.gpuHBMutil, gpuLeakage=serverTray.gpuLeakage, gpuNominalDieT=serverTray.gpuNominalDieT, gpuDieThermalC=serverTray.gpuDieThermalC_perGPU * itTray.nGPU(1), gpuHeatSinkR=serverTray.gpuHeatSinkR_perGPU / itTray.nGPU(1), gpuSurfArea=serverTray.gpuSurfArea_perGPU * itTray.nGPU(1), gpuAmbientR=serverTray.gpuAmbientR_perGPU / itTray.nGPU(1), nCPU=itTray.nCPU(1), cpuTDPperSocket=350, cpuIdlePower=80, cpuExponent=1.1, cpuLeakage=0.05, cpuNominalDieT=350, cpuDieThermalC=50, cpuHeatSinkR=0.15, cpuSurfArea=0.01, cpuAmbientR=0.5, initialT=serverTray.initialT, htc=serverTray.htc}
      mask prompts: nTrays "Number of IT trays per rack (-)"; nRacks "Number of racks (-)"; trayMass "Tray mass (kg)"; trayCp "Tray specific heat capacity (J/kg*K)"; trayThermalR "Tray to external thermal resistance (K/W)"; nGPU "Number of GPU per tray (-)"; gpuTDPperDie "GPU TDP per die (W)"; gpuIdlePower "GPU idle power (W)"; gpuHBMpower "HBM power per GPU (W)"; gpuExponent "GPU power utilization exponent (-)"; gpuHBMutil "HBM utilization as fraction of compute utilization (-)"; gpuLeakage "Leakage increase per K above nominal temperature (W/K)"; gpuNominalDieT "Nominal die temperature at TDP (K)"; gpuDieThermalC "GPU die thermal capacitance (J/K)"; gpuHeatSinkR "GPU die-heat-sink thermal resistance (K/W)"; gpuSurfArea "Surface area per die for ambient heat transfer (m^2)"; gpuAmbientR "GPU die-ambient thermal resistance (K/W)"; nCPU "Number of CPU per tray (-)"; cpuTDPperSocket "CPU TDP per socket (W)"; cpuIdlePower "CPU idle power per socket (W)"; cpuExponent "CPU power utilization exponent (-)"; cpuLeakage "Leakage increase per K above nominal temperature (W/K)"; cpuNominalDieT "Nominal die temperature at TDP (K)"; cpuDieThermalC "CPU die thermal capacitance (J/K)"; cpuHeatSinkR "CPU die-heat-sink thermal resistance (K/W)"; cpuSurfArea "Surface area per die for ambient heat transfer (m^2)"; cpuAmbientR "CPU die-ambient thermal resistance (K/W)"; initialT "Initial temperature (K)"; htc "Heat transfer coefficient to ambient (W/m^2.K)"
      settings: CopyFcn=set_param(gcbh,'LinkStatus','none');  PortSchema="{\"entries\":[{\"content\":{\"sides\":[{\"content\":{\"connectorIds\":[\"LConn1\",\"LConn2\",\"LConn3\"]},\"type\":\"ConnectorPlacement.EquallySpacedRectSide\",\"uuid\":\"1a9a884a-dab1-4495-bf62-c6b2de6c1039\"},{\"content\":{\"connectorIds\":[\"RConn1\",\"RConn2\",\"RConn3\"],\"side\":\"RIGHT\"},\"type\":\"ConnectorPlacement.EquallySpacedRectSide\",\"uuid\":\"05c53434-51c1-4fee-b885-c321dcda8b6b\"},{\"content\":{\"side\":\"TOP\"},\"type\":\"ConnectorPlacement.EquallySpacedRectSide\",\"uuid\":\"c7b5c534-d596-4858-a133-27f005e6c9d4\"},{\"content\":{\"connectorIds\":[\"RConn4\"],\"side\":\"BOTTOM\"},\"type\":\"ConnectorPlacement.EquallySpacedRectSide\",\"uuid\":\"693f3c99-4296-4d86-bfcc-da753d3e576f\"}]},\"type\":\"ConnectorPlacement.EquallySpacedConnector\",\"uuid\":\"ed91c467-c4d0-403f-af16-bac0257594fd\"}],\"packageUris\":[\"http://schema.mathworks.com/mf0/Connector/R2020b\"],\"version\":\"1.0\"}"
      mask Help: web("DocumentationPDURacks.html")
      mask DialogControl Container10 Prompt: PDU Racks
      mask DialogControl getRatingButton Prompt: Get Rating
      mask DialogControl Container9 Prompt: IT Tray
      mask DialogControl Container6 Prompt: GPU
      mask DialogControl Container7 Prompt: CPU
      mask DialogControl Container8 Prompt: Initial Conditions
      mask Display: image('icon_PDURacks.png');
  PS Gain : fl_lib/Physical Signals/Functions/PS Gain  gain=0.1
  PS Product : fl_lib/Physical Signals/Functions/PS Product
  PS-Simulink Converter : nesl_utility/PS-Simulink Converter  PhysicalDomain=network_engine_domain  SubClassName=ps_output  LeftPortType=input  RightPortType=output  PseudoPeriodic=off  Frequencies=[]  VectorFormat=inherit  Unit=inherit  AffineConversion=off
  PS-Simulink Converter1 : nesl_utility/PS-Simulink Converter  PhysicalDomain=network_engine_domain  SubClassName=ps_output  LeftPortType=input  RightPortType=output  PseudoPeriodic=off  Frequencies=[]  VectorFormat=inherit  Unit=inherit  AffineConversion=off
  PS-Simulink Converter2 : nesl_utility/PS-Simulink Converter  PhysicalDomain=network_engine_domain  SubClassName=ps_output  LeftPortType=input  RightPortType=output  PseudoPeriodic=off  Frequencies=[]  VectorFormat=inherit  Unit=inherit  AffineConversion=off
  Voltage Sensor : fl_lib/Electrical/Electrical Sensors/Voltage Sensor
  - : PMIOPort  Side=Left
  + : PMIOPort  Port=2  Side=Left
  U : PMIOPort  Port=3  Side=Left
  Pe : Outport
  TGPU : Outport  Port=2
  TCPU : Outport  Port=3
  wires:
  PS-Simulink Converter1/1 -> Pe/1
  PS-Simulink Converter/1 -> TGPU/1
  PS-Simulink Converter2/1 -> TCPU/1
  connections:
  DC-DC Converter/LConn2 -- Voltage Sensor/RConn2 -- -/RConn1 -- DC-DC Converter/RConn2 -- Electrical Reference/LConn1 -- " IT Load"/RConn1 -- Capacitor/RConn1
  Current Sensor/LConn1 -- Voltage Sensor/LConn1 -- +/RConn1
  PS-Simulink Converter1/LConn1 -- PS Product/RConn1
  Current Sensor/RConn2 -- DC-DC Converter/LConn1
  Current Sensor/RConn1 -- PS Product/LConn2
  Voltage Sensor/RConn1 -- PS Product/LConn1
  PS Gain/LConn1 -- U/RConn1 -- PDU Racks/LConn1
  PS Gain/RConn1 -- PDU Racks/LConn2
  PDU Racks/RConn2 -- PS-Simulink Converter/LConn1
  PDU Racks/RConn3 -- PS-Simulink Converter2/LConn1
  Capacitor/LConn1 -- DC-DC Converter/RConn1 -- " IT Load"/LConn1
  PDU Racks/RConn1 -- " IT Load"/LConn2

== system DataCenterStability/IT Load B ==
  " IT Load" : ee_lib/Passive/Dynamic Load  load_type=ee.enum.dc_ac.dc  min_supply_voltage=0.5 V  pow_min=1e-3 W  G_reverse=1e-6 S  deltaV=1e-3 V  f0=60 Hz  Vrms_min=200 V  tau=0.01 s  Vrms_ini=300 V  Vang_ini=0 deg
      settings: InternalSimscapePortConfiguration="{\"Bottom\":[],\"Left\":[{\"id\":\"p\",\"label\":\"+\",\"type\":\"foundation.electrical.electrical\"}],\"Right\":[{\"id\":\"n\",\"label\":\"-\",\"type\":\"foundation.electrical.electrical\"}],\"Top\":[{\"id\":\"P\",\"label\":\"P\",\"type\":\"input\"}]}"
  Capacitor : fl_lib/Electrical/Electrical Elements/Capacitor  c=1e-3 F  r=1e-4 Ohm  g=1e-6 1/Ohm  i_specify=off  i_priority=None  i=0 A  i_nominal_specify=off  i_nominal_value=1  i_nominal_unit=A  v_specify=off  v_priority=None  v=0 V  v_nominal_specify=off  v_nominal_value=1  v_nominal_unit=V  vc_specify=on  vc_priority=Low  vc=400 V  vc_nominal_specify=off  vc_nominal_value=1  vc_nominal_unit=V
  Current Sensor : fl_lib/Electrical/Electrical Sensors/Current Sensor
  DC-DC Converter : ee_lib/Semiconductors & Converters/Converters/DC-DC Converter  Vref_option=ee.enum.converters.voltageref.internal  v_ref=1 V  P_rated=itTray.dcdc.P_rated(2) MW  droop_enabled=false  droop_param=ee.enum.converters.droop.value  droop=0.1 V/A  droop_percent=2  Vref_droop=10 V  reversible=ee.enum.converters.directionality.unidirectional  G_diode=1e-8 1/Ohm  P_fixed=1 W  losses_option=ee.enum.converters.lossesOption.proportionalToSquaredCurrent  eff_rated=itTray.dcdc.eff * 100  tableOption=ee.enum.converters.lossTableOptionThermal.currentTemp  i_eff_vec=[-2, -1, 1, 2] A  v_eff_vec=[15, 30, 45] V  eff_vec=[66, 76, 80, 74]  eff_2D_table=[66, 66, 66; 76, 76, 76; 80, 80, 80; 74, 74, 74]  model_dynamics=ee.enum.converters.dynamics.no  tau=0.02 s  v_ini=10 V  v1_min=1 V  R1=1000 Ohm  R2=1000 Ohm  fault_condition=ee.enum.faults.faultInputCondition.greaterThan  fault_threshold=0.5  T_eff_vec=[280, 300, 320] K  eff_3D_table=repmat([66; 76; 80; 74], 1, 3, 3)  thermal_mass=100 J/K  initial_temperature=298.15 K
      settings: InternalSimscapePortConfiguration="{\"Bottom\":[],\"Left\":[{\"id\":\"p1\",\"label\":\"1+\",\"type\":\"foundation.electrical.electrical\"},{\"id\":\"n1\",\"label\":\"1-\",\"type\":\"foundation.electrical.electrical\"}],\"Right\":[{\"id\":\"p2\",\"label\":\"2+\",\"type\":\"foundation.electrical.electrical\"},{\"id\":\"n2\",\"label\":\"2-\",\"type\":\"foundation.electrical.electrical\"},{\"id\":\"H\",\"label\":\"H\",\"type\":\"foundation.thermal.thermal\"}],\"Top\":[]}"
  Electrical Reference : fl_lib/Electrical/Electrical Elements/Electrical Reference
  PDU Racks : Subsystem  mask{nTrays=36, nRacks=6, trayMass=serverTray.trayMass, trayCp=serverTray.trayCp, trayThermalR=serverTray.trayThermalR_perGPU / itTray.nGPU(2), nGPU=itTray.nGPU(2), gpuTDPperDie=serverTray.gpuTDPperDie, gpuIdlePower=serverTray.gpuIdlePower, gpuHBMpower=serverTray.gpuHBMpower, gpuExponent=serverTray.gpuExponent, gpuHBMutil=serverTray.gpuHBMutil, gpuLeakage=serverTray.gpuLeakage, gpuNominalDieT=serverTray.gpuNominalDieT, gpuDieThermalC=serverTray.gpuDieThermalC_perGPU * itTray.nGPU(2), gpuHeatSinkR=serverTray.gpuHeatSinkR_perGPU / itTray.nGPU(2), gpuSurfArea=serverTray.gpuSurfArea_perGPU * itTray.nGPU(2), gpuAmbientR=serverTray.gpuAmbientR_perGPU / itTray.nGPU(2), nCPU=itTray.nCPU(2), cpuTDPperSocket=350, cpuIdlePower=80, cpuExponent=1.1, cpuLeakage=0.05, cpuNominalDieT=350, cpuDieThermalC=50, cpuHeatSinkR=0.15, cpuSurfArea=0.01, cpuAmbientR=0.5, initialT=serverTray.initialT, htc=serverTray.htc}
      mask prompts: nTrays "Number of IT trays per rack (-)"; nRacks "Number of racks (-)"; trayMass "Tray mass (kg)"; trayCp "Tray specific heat capacity (J/kg*K)"; trayThermalR "Tray to external thermal resistance (K/W)"; nGPU "Number of GPU per tray (-)"; gpuTDPperDie "GPU TDP per die (W)"; gpuIdlePower "GPU idle power (W)"; gpuHBMpower "HBM power per GPU (W)"; gpuExponent "GPU power utilization exponent (-)"; gpuHBMutil "HBM utilization as fraction of compute utilization (-)"; gpuLeakage "Leakage increase per K above nominal temperature (W/K)"; gpuNominalDieT "Nominal die temperature at TDP (K)"; gpuDieThermalC "GPU die thermal capacitance (J/K)"; gpuHeatSinkR "GPU die-heat-sink thermal resistance (K/W)"; gpuSurfArea "Surface area per die for ambient heat transfer (m^2)"; gpuAmbientR "GPU die-ambient thermal resistance (K/W)"; nCPU "Number of CPU per tray (-)"; cpuTDPperSocket "CPU TDP per socket (W)"; cpuIdlePower "CPU idle power per socket (W)"; cpuExponent "CPU power utilization exponent (-)"; cpuLeakage "Leakage increase per K above nominal temperature (W/K)"; cpuNominalDieT "Nominal die temperature at TDP (K)"; cpuDieThermalC "CPU die thermal capacitance (J/K)"; cpuHeatSinkR "CPU die-heat-sink thermal resistance (K/W)"; cpuSurfArea "Surface area per die for ambient heat transfer (m^2)"; cpuAmbientR "CPU die-ambient thermal resistance (K/W)"; initialT "Initial temperature (K)"; htc "Heat transfer coefficient to ambient (W/m^2.K)"
      settings: CopyFcn=set_param(gcbh,'LinkStatus','none');  PortSchema="{\"entries\":[{\"content\":{\"sides\":[{\"content\":{\"connectorIds\":[\"LConn1\",\"LConn2\",\"LConn3\"]},\"type\":\"ConnectorPlacement.EquallySpacedRectSide\",\"uuid\":\"1a9a884a-dab1-4495-bf62-c6b2de6c1039\"},{\"content\":{\"connectorIds\":[\"RConn1\",\"RConn2\",\"RConn3\"],\"side\":\"RIGHT\"},\"type\":\"ConnectorPlacement.EquallySpacedRectSide\",\"uuid\":\"05c53434-51c1-4fee-b885-c321dcda8b6b\"},{\"content\":{\"side\":\"TOP\"},\"type\":\"ConnectorPlacement.EquallySpacedRectSide\",\"uuid\":\"c7b5c534-d596-4858-a133-27f005e6c9d4\"},{\"content\":{\"connectorIds\":[\"RConn4\"],\"side\":\"BOTTOM\"},\"type\":\"ConnectorPlacement.EquallySpacedRectSide\",\"uuid\":\"693f3c99-4296-4d86-bfcc-da753d3e576f\"}]},\"type\":\"ConnectorPlacement.EquallySpacedConnector\",\"uuid\":\"ed91c467-c4d0-403f-af16-bac0257594fd\"}],\"packageUris\":[\"http://schema.mathworks.com/mf0/Connector/R2020b\"],\"version\":\"1.0\"}"
      mask Help: web("DocumentationPDURacks.html")
      mask DialogControl Container10 Prompt: PDU Racks
      mask DialogControl getRatingButton Prompt: Get Rating
      mask DialogControl Container9 Prompt: IT Tray
      mask DialogControl Container6 Prompt: GPU
      mask DialogControl Container7 Prompt: CPU
      mask DialogControl Container8 Prompt: Initial Conditions
      mask Display: image('icon_PDURacks.png');
  PS Gain : fl_lib/Physical Signals/Functions/PS Gain  gain=0.1
  PS Product : fl_lib/Physical Signals/Functions/PS Product
  PS-Simulink Converter : nesl_utility/PS-Simulink Converter  PhysicalDomain=network_engine_domain  SubClassName=ps_output  LeftPortType=input  RightPortType=output  PseudoPeriodic=off  Frequencies=[]  VectorFormat=inherit  Unit=inherit  AffineConversion=off
  PS-Simulink Converter1 : nesl_utility/PS-Simulink Converter  PhysicalDomain=network_engine_domain  SubClassName=ps_output  LeftPortType=input  RightPortType=output  PseudoPeriodic=off  Frequencies=[]  VectorFormat=inherit  Unit=inherit  AffineConversion=off
  PS-Simulink Converter2 : nesl_utility/PS-Simulink Converter  PhysicalDomain=network_engine_domain  SubClassName=ps_output  LeftPortType=input  RightPortType=output  PseudoPeriodic=off  Frequencies=[]  VectorFormat=inherit  Unit=inherit  AffineConversion=off
  Voltage Sensor : fl_lib/Electrical/Electrical Sensors/Voltage Sensor
  - : PMIOPort  Side=Left
  + : PMIOPort  Port=2  Side=Left
  U : PMIOPort  Port=3  Side=Left
  Pe : Outport
  TGPU : Outport  Port=2
  TCPU : Outport  Port=3
  wires:
  PS-Simulink Converter1/1 -> Pe/1
  PS-Simulink Converter/1 -> TGPU/1
  PS-Simulink Converter2/1 -> TCPU/1
  connections:
  DC-DC Converter/RConn1 -- Capacitor/LConn1 -- " IT Load"/LConn1
  -/RConn1 -- Voltage Sensor/RConn2 -- DC-DC Converter/LConn2
  DC-DC Converter/RConn2 -- Electrical Reference/LConn1 -- " IT Load"/RConn1 -- Capacitor/RConn1
  +/RConn1 -- Voltage Sensor/LConn1 -- Current Sensor/LConn1
  PS-Simulink Converter1/LConn1 -- PS Product/RConn1
  Current Sensor/RConn2 -- DC-DC Converter/LConn1
  Current Sensor/RConn1 -- PS Product/LConn2
  Voltage Sensor/RConn1 -- PS Product/LConn1
  PS Gain/LConn1 -- U/RConn1 -- PDU Racks/LConn1
  PS Gain/RConn1 -- PDU Racks/LConn2
  PDU Racks/RConn1 -- " IT Load"/LConn2
  PDU Racks/RConn2 -- PS-Simulink Converter/LConn1
  PDU Racks/RConn3 -- PS-Simulink Converter2/LConn1
